simulink model "Regler_GUT"  (Simulink 7.4)
settings: Solver=ode45  StartTime=0.0  StopTime=15  RelTol=1e-3
values from neighbouring files (symbols this model uses):
  K_ret = place(System.a, System.b, [-18 -5 -7 -10 -9])    [Test_Reglerauslegung.m]
  KV = KV'    [Reglerauslegung.m]    (also in Test_Reglerauslegung.m)
  phi0 = 0.15    [Quadrocopter_control_Driver.m]    (also in calc_stability.m = 0)
  r_psi0 = 0    [Quadrocopter_control_Driver.m]    (also in calc_stability.m)
  r_theta0 = 0    [Quadrocopter_control_Driver.m]    (also in calc_stability.m)
  theta0 = 0.15    [Quadrocopter_control_Driver.m]    (also in calc_stability.m = 0)
undefined symbols (not defined in the file or in its folder): boom, f1, f2, f3, f4, f5, I_x, I_y, I_z
libraries: Copter_Library x5
settings Model: Creator=alstit04  LastModifiedBy=Alex

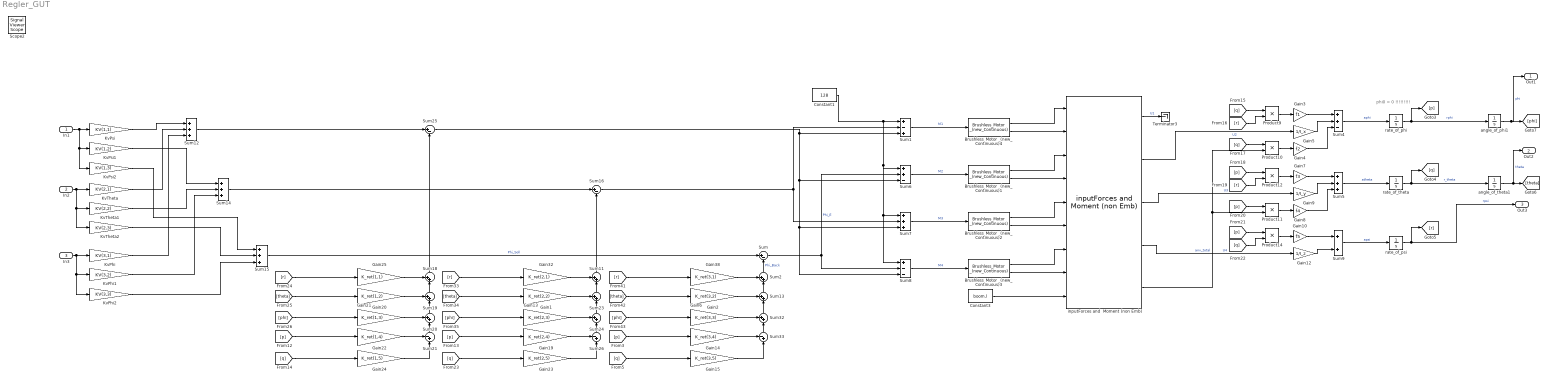
== system Regler_GUT ==
  note: phi0 = 0 !!!!!!!!!
  In1 : Inport  OutDataType=fixdt(1, 16)  OutScaling=2^0
  In2 : Inport  Port=2  OutDataType=fixdt(1, 16)  OutScaling=2^0
  In3 : Inport  Port=3  OutDataType=fixdt(1, 16)  OutScaling=2^0
  Brushless_Motor _(new_Continuous){1..4} (4 alike) : Copter_Library/Brushless_Motor _(new_Continuous)  SystemSampleTime=-1  M_error=0.99
  Constant1 : Constant  Value=128
  Constant3 : Constant  Value=boom.l
  Gain1 : Gain  Gain=K_ret(2,2)  ParameterDataType=fixdt(1, 16)  ParameterScaling=2^0  OutDataType=fixdt(1, 16)  OutScaling=2^0
  Gain10 : Gain  Gain=f5
  Gain12 : Gain  Gain=1/I_z
  Gain13 : Gain  Gain=K_ret(2,3)  ParameterDataType=fixdt(1, 16)  ParameterScaling=2^0  OutDataType=fixdt(1, 16)  OutScaling=2^0
  Gain14 : Gain  Gain=K_ret(3,4)  ParameterDataType=fixdt(1, 16)  ParameterScaling=2^0  OutDataType=fixdt(1, 16)  OutScaling=2^0
  Gain15 : Gain  Gain=K_ret(3,5)  ParameterDataType=fixdt(1, 16)  ParameterScaling=2^0  OutDataType=fixdt(1, 16)  OutScaling=2^0
  Gain19 : Gain  Gain=K_ret(2,4)  ParameterDataType=fixdt(1, 16)  ParameterScaling=2^0  OutDataType=fixdt(1, 16)  OutScaling=2^0
  Gain2 : Gain  Gain=K_ret(3,2)  ParameterDataType=fixdt(1, 16)  ParameterScaling=2^0  OutDataType=fixdt(1, 16)  OutScaling=2^0
  Gain20 : Gain  Gain=K_ret(1,2)  ParameterDataType=fixdt(1, 16)  ParameterScaling=2^0  OutDataType=fixdt(1, 16)  OutScaling=2^0
  Gain21 : Gain  Gain=K_ret(1,3)  ParameterDataType=fixdt(1, 16)  ParameterScaling=2^0  OutDataType=fixdt(1, 16)  OutScaling=2^0
  Gain22 : Gain  Gain=K_ret(1,4)  ParameterDataType=fixdt(1, 16)  ParameterScaling=2^0  OutDataType=fixdt(1, 16)  OutScaling=2^0
  Gain23 : Gain  Gain=K_ret(2,5)  ParameterDataType=fixdt(1, 16)  ParameterScaling=2^0  OutDataType=fixdt(1, 16)  OutScaling=2^0
  Gain24 : Gain  Gain=K_ret(1,5)  ParameterDataType=fixdt(1, 16)  ParameterScaling=2^0  OutDataType=fixdt(1, 16)  OutScaling=2^0
  Gain25 : Gain  Gain=K_ret(1,1)  ParameterDataType=fixdt(1, 16)  ParameterScaling=2^0  OutDataType=fixdt(1, 16)  OutScaling=2^0
  Gain3 : Gain  Gain=f1
  Gain32 : Gain  Gain=K_ret(2,1)  ParameterDataType=fixdt(1, 16)  ParameterScaling=2^0  OutDataType=fixdt(1, 16)  OutScaling=2^0
  Gain38 : Gain  Gain=K_ret(3,1)  ParameterDataType=fixdt(1, 16)  ParameterScaling=2^0  OutDataType=fixdt(1, 16)  OutScaling=2^0
  Gain4 : Gain  Gain=f2
  Gain5 : Gain  Gain=1/I_x
  Gain6 : Gain  Gain=K_ret(3,3)  ParameterDataType=fixdt(1, 16)  ParameterScaling=2^0  OutDataType=fixdt(1, 16)  OutScaling=2^0
  Gain7 : Gain  Gain=f3
  Gain8 : Gain  Gain=f4
  Gain9 : Gain  Gain=1/I_y
  KvPhi : Gain  Gain=KV(3,1)  ParameterDataType=fixdt(1, 16)  ParameterScaling=2^0  OutDataType=fixdt(1, 16)  OutScaling=2^0
  KvPhi1 : Gain  Gain=KV(3,2)  ParameterDataType=fixdt(1, 16)  ParameterScaling=2^0  OutDataType=fixdt(1, 16)  OutScaling=2^0
  KvPhi2 : Gain  Gain=KV(3,3)  ParameterDataType=fixdt(1, 16)  ParameterScaling=2^0  OutDataType=fixdt(1, 16)  OutScaling=2^0
  KvPsi : Gain  Gain=KV(1,1)  ParameterDataType=fixdt(1, 16)  ParameterScaling=2^0  OutDataType=fixdt(1, 16)  OutScaling=2^0
  KvPsi1 : Gain  Gain=KV(1,2)  ParameterDataType=fixdt(1, 16)  ParameterScaling=2^0  OutDataType=fixdt(1, 16)  OutScaling=2^0
  KvPsi2 : Gain  Gain=KV(1,3)  ParameterDataType=fixdt(1, 16)  ParameterScaling=2^0  OutDataType=fixdt(1, 16)  OutScaling=2^0
  KvTheta : Gain  Gain=KV(2,1)  ParameterDataType=fixdt(1, 16)  ParameterScaling=2^0  OutDataType=fixdt(1, 16)  OutScaling=2^0
  KvTheta1 : Gain  Gain=KV(2,2)  ParameterDataType=fixdt(1, 16)  ParameterScaling=2^0  OutDataType=fixdt(1, 16)  OutScaling=2^0
  KvTheta2 : Gain  Gain=KV(2,3)  ParameterDataType=fixdt(1, 16)  ParameterScaling=2^0  OutDataType=fixdt(1, 16)  OutScaling=2^0
  Product{9..12,14} (5 alike) : Product  RndMeth=Zero
  Sum : Sum  Inputs=|+-  OutDataType=fixdt(1, 16)  OutScaling=2^0
  Sum1 : Sum  Inputs=+-+  OutDataType=fixdt(1, 16)  OutScaling=2^0
  Sum{2,11,13,18..20,23..24,32} (9 alike) : Sum  Inputs=++|  OutDataType=fixdt(1, 16)  OutScaling=2^0
  Sum{7,12,14..15} (4 alike) : Sum  Inputs=+++  OutDataType=fixdt(1, 16)  OutScaling=2^0
  Sum16 : Sum  Inputs=|+-  OutDataType=fixdt(1, 16)  OutScaling=2^0
  Sum21 : Sum  Inputs=-+|  OutDataType=fixdt(1, 16)  OutScaling=2^0
  Sum25 : Sum  Inputs=|+-  OutDataType=fixdt(1, 16)  OutScaling=2^0
  Sum26 : Sum  Inputs=-+|  OutDataType=fixdt(1, 16)  OutScaling=2^0
  Sum33 : Sum  Inputs=-+|  OutDataType=fixdt(1, 16)  OutScaling=2^0
  Sum4 : Sum  Inputs=++-
  Sum5 : Sum  Inputs=+++
  Sum6 : Sum  Inputs=++-  OutDataType=fixdt(1, 16)  OutScaling=2^0
  Sum8 : Sum  Inputs=+--  OutDataType=fixdt(1, 16)  OutScaling=2^0
  Sum9 : Sum
  Terminator3 : Terminator
  angle_of_phi1 : Integrator  InitialCondition=phi0
  angle_of_theta1 : Integrator  InitialCondition=theta0
  inputForces and  Moment (non Emb) : Copter_Library/inputForces and  Moment (non Emb)  SystemSampleTime=-1
  rate_of_phi : Integrator
  rate_of_psi : Integrator  InitialCondition=r_psi0
  rate_of_theta : Integrator  InitialCondition=r_theta0
  Out1 : Outport  OutDataType=fixdt(1, 16)  OutScaling=2^0
  Out2 : Outport  Port=2  OutDataType=fixdt(1, 16)  OutScaling=2^0
  Out3 : Outport  Port=3  OutDataType=fixdt(1, 16)  OutScaling=2^0
  Scope2 : SignalViewerScope  IOType=viewer  NumInputPorts=3  RefreshTime=0.035000
      settings: ShowLegends=on  TimeRange=15  YMin=-1~-0.2~-5  YMax=1~1.2~5  SaveToWorkspace=on
  wires:
  Sum8/1 -> Brushless_Motor _(new_Continuous)3/1  "M4"
  Sum6/1 -> Brushless_Motor _(new_Continuous)1/1  "M2"
  Sum1/1 -> Brushless_Motor _(new_Continuous)4/1  "M1"
  Constant1/1 -> Sum1/1, Sum6/1, Sum7/1, Sum8/1
  Sum7/1 -> Brushless_Motor _(new_Continuous)2/1  "M3"
  Constant3/1 -> inputForces and  Moment (non Emb)/9
  Sum9/1 -> rate_of_psi/1  "apsi"
  inputForces and  Moment (non Emb)/4 -> Gain12/1  "U4"
  Gain12/1 -> Sum9/2
  Gain10/1 -> Sum9/1
  Product14/1 -> Gain10/1
  [q] -> Product14/2
  [p] -> Product14/1
  Sum5/1 -> rate_of_theta/1  "atheta"
  inputForces and  Moment (non Emb)/3 -> Gain9/1  "U3"
  Gain8/1 -> Sum5/3
  Gain9/1 -> Sum5/2
  Product11/1 -> Gain8/1
  [p] -> Product11/1
  Gain7/1 -> Sum5/1
  Product12/1 -> Gain7/1
  [r] -> Product12/2
  [p] -> Product12/1
  Sum4/1 -> rate_of_phi/1  "aphi"
  Gain4/1 -> Sum4/3
  Gain5/1 -> Sum4/2
  inputForces and  Moment (non Emb)/2 -> Gain5/1  "U2"
  Product10/1 -> Gain4/1
  [q] -> Product10/1
  Gain3/1 -> Sum4/1
  Product9/1 -> Gain3/1
  [r] -> Product9/2
  [q] -> Product9/1
  inputForces and  Moment (non Emb)/5 -> Product11/2, Product10/2  "anv_total"
  rate_of_phi/1 -> [p], angle_of_phi1/1  "rphi"
  rate_of_theta/1 -> [q], angle_of_theta1/1  "r_theta"
  rate_of_psi/1 -> [r], Out3/1  "rpsi"
  Brushless_Motor _(new_Continuous)4/1 -> inputForces and  Moment (non Emb)/1
  Brushless_Motor _(new_Continuous)4/2 -> inputForces and  Moment (non Emb)/2
  Brushless_Motor _(new_Continuous)1/1 -> inputForces and  Moment (non Emb)/3
  Brushless_Motor _(new_Continuous)1/2 -> inputForces and  Moment (non Emb)/4
  Brushless_Motor _(new_Continuous)2/1 -> inputForces and  Moment (non Emb)/5
  Brushless_Motor _(new_Continuous)2/2 -> inputForces and  Moment (non Emb)/6
  Brushless_Motor _(new_Continuous)3/1 -> inputForces and  Moment (non Emb)/7
  Brushless_Motor _(new_Continuous)3/2 -> inputForces and  Moment (non Emb)/8
  Sum/1 -> Sum6/2, Sum8/2  "Phi_E"
  Sum14/1 -> Sum16/1
  angle_of_phi1/1 -> [phi], Out1/1  "phi"
  angle_of_theta1/1 -> [theta], Out2/1  "theta"
  [r] -> Gain32/1
  [theta] -> Gain1/1
  [phi] -> Gain13/1
  Sum11/1 -> Sum16/2
  Gain1/1 -> Sum23/1
  Sum24/1 -> Sum23/2
  Sum23/1 -> Sum11/2
  [p] -> Gain19/1
  Sum26/1 -> Sum24/2
  [q] -> Gain23/1
  Gain23/1 -> Sum26/2
  [r] -> Gain38/1
  [theta] -> Gain2/1
  [phi] -> Gain6/1
  Sum2/1 -> Sum/2  "Phi_Back"
  Sum32/1 -> Sum13/2
  Sum13/1 -> Sum2/2
  [p] -> Gain14/1
  Sum33/1 -> Sum32/2
  [q] -> Gain15/1
  Sum25/1 -> Sum1/3, Sum6/3, Sum8/3, Sum7/3
  Sum16/1 -> Sum1/2, Sum7/2
  inputForces and  Moment (non Emb)/1 -> Terminator3/1  "U1"
  Gain19/1 -> Sum26/1
  Gain13/1 -> Sum24/1
  Gain32/1 -> Sum11/1
  Sum15/1 -> Sum/1  "Phi_Soll"
  Gain38/1 -> Sum2/1
  Gain2/1 -> Sum13/1
  Gain6/1 -> Sum32/1
  Gain14/1 -> Sum33/1
  Gain15/1 -> Sum33/2
  [r] -> Gain25/1
  [theta] -> Gain20/1
  [phi] -> Gain21/1
  Gain25/1 -> Sum18/1
  Sum20/1 -> Sum19/2
  Sum19/1 -> Sum18/2
  [p] -> Gain22/1
  Sum21/1 -> Sum20/2
  [q] -> Gain24/1
  Gain24/1 -> Sum21/2
  Gain22/1 -> Sum21/1
  Gain21/1 -> Sum20/1
  Gain20/1 -> Sum19/1
  Sum18/1 -> Sum25/2
  KvPsi/1 -> Sum12/1
  KvTheta/1 -> Sum12/2
  Sum12/1 -> Sum25/1
  KvPhi/1 -> Sum12/3
  KvPsi1/1 -> Sum14/1
  KvTheta1/1 -> Sum14/2
  KvPhi1/1 -> Sum14/3
  KvPhi2/1 -> Sum15/3
  KvTheta2/1 -> Sum15/2
  KvPsi2/1 -> Sum15/1
  In1/1 -> KvPsi/1, KvPsi1/1, KvPsi2/1
  In2/1 -> KvTheta/1, KvTheta1/1, KvTheta2/1
  In3/1 -> KvPhi/1, KvPhi1/1, KvPhi2/1
